simulink model "gm_hybrid_lht_vnl"  (R2019b)
settings: Solver=FixedStepDiscrete  StartTime=0.0  StopTime=inf  FixedStep=1/120e6  RelTol=1e-3
undefined symbols (not defined in the file or in its folder): bt, height, nTheta, width
libraries: hdlsllib x252, simulink x168, hdlmdlgenlib x11, dspsrcs4 x1
(part 8 of 12)

== system gm_hybrid_lht_vnl/Hybrid LHT/Hybrid LHT Kernel/Gradient Kernel System/Get Index and Fix Limits/GetShift1_instance25 ==
  Theta : Inport  OutDataTypeStr=uint8  PortDimensions=1  SampleTime=8.33333333333333e-09
  Add : Sum  Inputs=+  OutDataTypeStr=fixdt(0, ceil(log2(L+1)), 0)
  Constant : Constant  Value=U  VectorParams1D=off  OutDataTypeStr=fixdt(0,ceil(log2(max(U)+1)),0)  SampleTime=-1
  Relational Operator : RelationalOperator  OutDataTypeStr=boolean  RndMeth=Nearest
  Shift : Outport  VectorParamsAs1DForOutWhenUnconnected=off
  wires:
  Relational Operator/1 -> Add/1
  Constant/1 -> Relational Operator/2
  Add/1 -> Shift/1
  Theta/1 -> Relational Operator/1

== system gm_hybrid_lht_vnl/Hybrid LHT/Hybrid LHT Kernel/Gradient Kernel System/Get Index and Fix Limits/GetShift1_instance26 ==
  Theta : Inport  OutDataTypeStr=uint8  PortDimensions=1  SampleTime=8.33333333333333e-09
  Add : Sum  Inputs=+  OutDataTypeStr=fixdt(0, ceil(log2(L+1)), 0)
  Constant : Constant  Value=U  VectorParams1D=off  OutDataTypeStr=fixdt(0,ceil(log2(max(U)+1)),0)  SampleTime=-1
  Relational Operator : RelationalOperator  OutDataTypeStr=boolean  RndMeth=Nearest
  Shift : Outport  VectorParamsAs1DForOutWhenUnconnected=off
  wires:
  Relational Operator/1 -> Add/1
  Constant/1 -> Relational Operator/2
  Add/1 -> Shift/1
  Theta/1 -> Relational Operator/1

== system gm_hybrid_lht_vnl/Hybrid LHT/Hybrid LHT Kernel/Gradient Kernel System/Get Index and Fix Limits/GetShift1_instance27 ==
  Theta : Inport  OutDataTypeStr=uint8  PortDimensions=1  SampleTime=8.33333333333333e-09
  Add : Sum  Inputs=+  OutDataTypeStr=fixdt(0, ceil(log2(L+1)), 0)
  Constant : Constant  Value=U  VectorParams1D=off  OutDataTypeStr=fixdt(0,ceil(log2(max(U)+1)),0)  SampleTime=-1
  Relational Operator : RelationalOperator  OutDataTypeStr=boolean  RndMeth=Nearest
  Shift : Outport  VectorParamsAs1DForOutWhenUnconnected=off
  wires:
  Relational Operator/1 -> Add/1
  Constant/1 -> Relational Operator/2
  Add/1 -> Shift/1
  Theta/1 -> Relational Operator/1

== system gm_hybrid_lht_vnl/Hybrid LHT/Hybrid LHT Kernel/Gradient Kernel System/Get Index and Fix Limits/GetShift1_instance28 ==
  Theta : Inport  OutDataTypeStr=uint8  PortDimensions=1  SampleTime=8.33333333333333e-09
  Add : Sum  Inputs=+  OutDataTypeStr=fixdt(0, ceil(log2(L+1)), 0)
  Constant : Constant  Value=U  VectorParams1D=off  OutDataTypeStr=fixdt(0,ceil(log2(max(U)+1)),0)  SampleTime=-1
  Relational Operator : RelationalOperator  OutDataTypeStr=boolean  RndMeth=Nearest
  Shift : Outport  VectorParamsAs1DForOutWhenUnconnected=off
  wires:
  Relational Operator/1 -> Add/1
  Constant/1 -> Relational Operator/2
  Add/1 -> Shift/1
  Theta/1 -> Relational Operator/1

== system gm_hybrid_lht_vnl/Hybrid LHT/Hybrid LHT Kernel/Gradient Kernel System/Get Index and Fix Limits/GetShift1_instance29 ==
  Theta : Inport  OutDataTypeStr=uint8  PortDimensions=1  SampleTime=8.33333333333333e-09
  Add : Sum  Inputs=+  OutDataTypeStr=fixdt(0, ceil(log2(L+1)), 0)
  Constant : Constant  Value=U  VectorParams1D=off  OutDataTypeStr=fixdt(0,ceil(log2(max(U)+1)),0)  SampleTime=-1
  Relational Operator : RelationalOperator  OutDataTypeStr=boolean  RndMeth=Nearest
  Shift : Outport  VectorParamsAs1DForOutWhenUnconnected=off
  wires:
  Relational Operator/1 -> Add/1
  Constant/1 -> Relational Operator/2
  Add/1 -> Shift/1
  Theta/1 -> Relational Operator/1

== system gm_hybrid_lht_vnl/Hybrid LHT/Hybrid LHT Kernel/Gradient Kernel System/Get Index and Fix Limits/GetShift1_instance3 ==
  Theta : Inport  OutDataTypeStr=uint8  PortDimensions=1  SampleTime=8.33333333333333e-09
  Add : Sum  Inputs=+  OutDataTypeStr=fixdt(0, ceil(log2(L+1)), 0)
  Constant : Constant  Value=U  VectorParams1D=off  OutDataTypeStr=fixdt(0,ceil(log2(max(U)+1)),0)  SampleTime=-1
  Relational Operator : RelationalOperator  OutDataTypeStr=boolean  RndMeth=Nearest
  Shift : Outport  VectorParamsAs1DForOutWhenUnconnected=off
  wires:
  Relational Operator/1 -> Add/1
  Constant/1 -> Relational Operator/2
  Add/1 -> Shift/1
  Theta/1 -> Relational Operator/1

== system gm_hybrid_lht_vnl/Hybrid LHT/Hybrid LHT Kernel/Gradient Kernel System/Get Index and Fix Limits/GetShift1_instance30 ==
  Theta : Inport  OutDataTypeStr=uint8  PortDimensions=1  SampleTime=8.33333333333333e-09
  Add : Sum  Inputs=+  OutDataTypeStr=fixdt(0, ceil(log2(L+1)), 0)
  Constant : Constant  Value=U  VectorParams1D=off  OutDataTypeStr=fixdt(0,ceil(log2(max(U)+1)),0)  SampleTime=-1
  Relational Operator : RelationalOperator  OutDataTypeStr=boolean  RndMeth=Nearest
  Shift : Outport  VectorParamsAs1DForOutWhenUnconnected=off
  wires:
  Relational Operator/1 -> Add/1
  Constant/1 -> Relational Operator/2
  Add/1 -> Shift/1
  Theta/1 -> Relational Operator/1

== system gm_hybrid_lht_vnl/Hybrid LHT/Hybrid LHT Kernel/Gradient Kernel System/Get Index and Fix Limits/GetShift1_instance31 ==
  Theta : Inport  OutDataTypeStr=uint8  PortDimensions=1  SampleTime=8.33333333333333e-09
  Add : Sum  Inputs=+  OutDataTypeStr=fixdt(0, ceil(log2(L+1)), 0)
  Constant : Constant  Value=U  VectorParams1D=off  OutDataTypeStr=fixdt(0,ceil(log2(max(U)+1)),0)  SampleTime=-1
  Relational Operator : RelationalOperator  OutDataTypeStr=boolean  RndMeth=Nearest
  Shift : Outport  VectorParamsAs1DForOutWhenUnconnected=off
  wires:
  Relational Operator/1 -> Add/1
  Constant/1 -> Relational Operator/2
  Add/1 -> Shift/1
  Theta/1 -> Relational Operator/1

== system gm_hybrid_lht_vnl/Hybrid LHT/Hybrid LHT Kernel/Gradient Kernel System/Get Index and Fix Limits/GetShift1_instance32 ==
  Theta : Inport  OutDataTypeStr=uint8  PortDimensions=1  SampleTime=8.33333333333333e-09
  Add : Sum  Inputs=+  OutDataTypeStr=fixdt(0, ceil(log2(L+1)), 0)
  Constant : Constant  Value=U  VectorParams1D=off  OutDataTypeStr=fixdt(0,ceil(log2(max(U)+1)),0)  SampleTime=-1
  Relational Operator : RelationalOperator  OutDataTypeStr=boolean  RndMeth=Nearest
  Shift : Outport  VectorParamsAs1DForOutWhenUnconnected=off
  wires:
  Relational Operator/1 -> Add/1
  Constant/1 -> Relational Operator/2
  Add/1 -> Shift/1
  Theta/1 -> Relational Operator/1

== system gm_hybrid_lht_vnl/Hybrid LHT/Hybrid LHT Kernel/Gradient Kernel System/Get Index and Fix Limits/GetShift1_instance33 ==
  Theta : Inport  OutDataTypeStr=uint8  PortDimensions=1  SampleTime=8.33333333333333e-09
  Add : Sum  Inputs=+  OutDataTypeStr=fixdt(0, ceil(log2(L+1)), 0)
  Constant : Constant  Value=U  VectorParams1D=off  OutDataTypeStr=fixdt(0,ceil(log2(max(U)+1)),0)  SampleTime=-1
  Relational Operator : RelationalOperator  OutDataTypeStr=boolean  RndMeth=Nearest
  Shift : Outport  VectorParamsAs1DForOutWhenUnconnected=off
  wires:
  Relational Operator/1 -> Add/1
  Constant/1 -> Relational Operator/2
  Add/1 -> Shift/1
  Theta/1 -> Relational Operator/1

== system gm_hybrid_lht_vnl/Hybrid LHT/Hybrid LHT Kernel/Gradient Kernel System/Get Index and Fix Limits/GetShift1_instance34 ==
  Theta : Inport  OutDataTypeStr=uint8  PortDimensions=1  SampleTime=8.33333333333333e-09
  Add : Sum  Inputs=+  OutDataTypeStr=fixdt(0, ceil(log2(L+1)), 0)
  Constant : Constant  Value=U  VectorParams1D=off  OutDataTypeStr=fixdt(0,ceil(log2(max(U)+1)),0)  SampleTime=-1
  Relational Operator : RelationalOperator  OutDataTypeStr=boolean  RndMeth=Nearest
  Shift : Outport  VectorParamsAs1DForOutWhenUnconnected=off
  wires:
  Relational Operator/1 -> Add/1
  Constant/1 -> Relational Operator/2
  Add/1 -> Shift/1
  Theta/1 -> Relational Operator/1

== system gm_hybrid_lht_vnl/Hybrid LHT/Hybrid LHT Kernel/Gradient Kernel System/Get Index and Fix Limits/GetShift1_instance35 ==
  Theta : Inport  OutDataTypeStr=uint8  PortDimensions=1  SampleTime=8.33333333333333e-09
  Add : Sum  Inputs=+  OutDataTypeStr=fixdt(0, ceil(log2(L+1)), 0)
  Constant : Constant  Value=U  VectorParams1D=off  OutDataTypeStr=fixdt(0,ceil(log2(max(U)+1)),0)  SampleTime=-1
  Relational Operator : RelationalOperator  OutDataTypeStr=boolean  RndMeth=Nearest
  Shift : Outport  VectorParamsAs1DForOutWhenUnconnected=off
  wires:
  Relational Operator/1 -> Add/1
  Constant/1 -> Relational Operator/2
  Add/1 -> Shift/1
  Theta/1 -> Relational Operator/1

== system gm_hybrid_lht_vnl/Hybrid LHT/Hybrid LHT Kernel/Gradient Kernel System/Get Index and Fix Limits/GetShift1_instance36 ==
  Theta : Inport  OutDataTypeStr=uint8  PortDimensions=1  SampleTime=8.33333333333333e-09
  Add : Sum  Inputs=+  OutDataTypeStr=fixdt(0, ceil(log2(L+1)), 0)
  Constant : Constant  Value=U  VectorParams1D=off  OutDataTypeStr=fixdt(0,ceil(log2(max(U)+1)),0)  SampleTime=-1
  Relational Operator : RelationalOperator  OutDataTypeStr=boolean  RndMeth=Nearest
  Shift : Outport  VectorParamsAs1DForOutWhenUnconnected=off
  wires:
  Relational Operator/1 -> Add/1
  Constant/1 -> Relational Operator/2
  Add/1 -> Shift/1
  Theta/1 -> Relational Operator/1

== system gm_hybrid_lht_vnl/Hybrid LHT/Hybrid LHT Kernel/Gradient Kernel System/Get Index and Fix Limits/GetShift1_instance37 ==
  Theta : Inport  OutDataTypeStr=uint8  PortDimensions=1  SampleTime=8.33333333333333e-09
  Add : Sum  Inputs=+  OutDataTypeStr=fixdt(0, ceil(log2(L+1)), 0)
  Constant : Constant  Value=U  VectorParams1D=off  OutDataTypeStr=fixdt(0,ceil(log2(max(U)+1)),0)  SampleTime=-1
  Relational Operator : RelationalOperator  OutDataTypeStr=boolean  RndMeth=Nearest
  Shift : Outport  VectorParamsAs1DForOutWhenUnconnected=off
  wires:
  Relational Operator/1 -> Add/1
  Constant/1 -> Relational Operator/2
  Add/1 -> Shift/1
  Theta/1 -> Relational Operator/1

== system gm_hybrid_lht_vnl/Hybrid LHT/Hybrid LHT Kernel/Gradient Kernel System/Get Index and Fix Limits/GetShift1_instance38 ==
  Theta : Inport  OutDataTypeStr=uint8  PortDimensions=1  SampleTime=8.33333333333333e-09
  Add : Sum  Inputs=+  OutDataTypeStr=fixdt(0, ceil(log2(L+1)), 0)
  Constant : Constant  Value=U  VectorParams1D=off  OutDataTypeStr=fixdt(0,ceil(log2(max(U)+1)),0)  SampleTime=-1
  Relational Operator : RelationalOperator  OutDataTypeStr=boolean  RndMeth=Nearest
  Shift : Outport  VectorParamsAs1DForOutWhenUnconnected=off
  wires:
  Relational Operator/1 -> Add/1
  Constant/1 -> Relational Operator/2
  Add/1 -> Shift/1
  Theta/1 -> Relational Operator/1

== system gm_hybrid_lht_vnl/Hybrid LHT/Hybrid LHT Kernel/Gradient Kernel System/Get Index and Fix Limits/GetShift1_instance39 ==
  Theta : Inport  OutDataTypeStr=uint8  PortDimensions=1  SampleTime=8.33333333333333e-09
  Add : Sum  Inputs=+  OutDataTypeStr=fixdt(0, ceil(log2(L+1)), 0)
  Constant : Constant  Value=U  VectorParams1D=off  OutDataTypeStr=fixdt(0,ceil(log2(max(U)+1)),0)  SampleTime=-1
  Relational Operator : RelationalOperator  OutDataTypeStr=boolean  RndMeth=Nearest
  Shift : Outport  VectorParamsAs1DForOutWhenUnconnected=off
  wires:
  Relational Operator/1 -> Add/1
  Constant/1 -> Relational Operator/2
  Add/1 -> Shift/1
  Theta/1 -> Relational Operator/1

== system gm_hybrid_lht_vnl/Hybrid LHT/Hybrid LHT Kernel/Gradient Kernel System/Get Index and Fix Limits/GetShift1_instance4 ==
  Theta : Inport  OutDataTypeStr=uint8  PortDimensions=1  SampleTime=8.33333333333333e-09
  Add : Sum  Inputs=+  OutDataTypeStr=fixdt(0, ceil(log2(L+1)), 0)
  Constant : Constant  Value=U  VectorParams1D=off  OutDataTypeStr=fixdt(0,ceil(log2(max(U)+1)),0)  SampleTime=-1
  Relational Operator : RelationalOperator  OutDataTypeStr=boolean  RndMeth=Nearest
  Shift : Outport  VectorParamsAs1DForOutWhenUnconnected=off
  wires:
  Relational Operator/1 -> Add/1
  Constant/1 -> Relational Operator/2
  Add/1 -> Shift/1
  Theta/1 -> Relational Operator/1

== system gm_hybrid_lht_vnl/Hybrid LHT/Hybrid LHT Kernel/Gradient Kernel System/Get Index and Fix Limits/GetShift1_instance40 ==
  Theta : Inport  OutDataTypeStr=uint8  PortDimensions=1  SampleTime=8.33333333333333e-09
  Add : Sum  Inputs=+  OutDataTypeStr=fixdt(0, ceil(log2(L+1)), 0)
  Constant : Constant  Value=U  VectorParams1D=off  OutDataTypeStr=fixdt(0,ceil(log2(max(U)+1)),0)  SampleTime=-1
  Relational Operator : RelationalOperator  OutDataTypeStr=boolean  RndMeth=Nearest
  Shift : Outport  VectorParamsAs1DForOutWhenUnconnected=off
  wires:
  Relational Operator/1 -> Add/1
  Constant/1 -> Relational Operator/2
  Add/1 -> Shift/1
  Theta/1 -> Relational Operator/1

== system gm_hybrid_lht_vnl/Hybrid LHT/Hybrid LHT Kernel/Gradient Kernel System/Get Index and Fix Limits/GetShift1_instance41 ==
  Theta : Inport  OutDataTypeStr=uint8  PortDimensions=1  SampleTime=8.33333333333333e-09
  Add : Sum  Inputs=+  OutDataTypeStr=fixdt(0, ceil(log2(L+1)), 0)
  Constant : Constant  Value=U  VectorParams1D=off  OutDataTypeStr=fixdt(0,ceil(log2(max(U)+1)),0)  SampleTime=-1
  Relational Operator : RelationalOperator  OutDataTypeStr=boolean  RndMeth=Nearest
  Shift : Outport  VectorParamsAs1DForOutWhenUnconnected=off
  wires:
  Relational Operator/1 -> Add/1
  Constant/1 -> Relational Operator/2
  Add/1 -> Shift/1
  Theta/1 -> Relational Operator/1

== system gm_hybrid_lht_vnl/Hybrid LHT/Hybrid LHT Kernel/Gradient Kernel System/Get Index and Fix Limits/GetShift1_instance42 ==
  Theta : Inport  OutDataTypeStr=uint8  PortDimensions=1  SampleTime=8.33333333333333e-09
  Add : Sum  Inputs=+  OutDataTypeStr=fixdt(0, ceil(log2(L+1)), 0)
  Constant : Constant  Value=U  VectorParams1D=off  OutDataTypeStr=fixdt(0,ceil(log2(max(U)+1)),0)  SampleTime=-1
  Relational Operator : RelationalOperator  OutDataTypeStr=boolean  RndMeth=Nearest
  Shift : Outport  VectorParamsAs1DForOutWhenUnconnected=off
  wires:
  Relational Operator/1 -> Add/1
  Constant/1 -> Relational Operator/2
  Add/1 -> Shift/1
  Theta/1 -> Relational Operator/1

== system gm_hybrid_lht_vnl/Hybrid LHT/Hybrid LHT Kernel/Gradient Kernel System/Get Index and Fix Limits/GetShift1_instance43 ==
  Theta : Inport  OutDataTypeStr=uint8  PortDimensions=1  SampleTime=8.33333333333333e-09
  Add : Sum  Inputs=+  OutDataTypeStr=fixdt(0, ceil(log2(L+1)), 0)
  Constant : Constant  Value=U  VectorParams1D=off  OutDataTypeStr=fixdt(0,ceil(log2(max(U)+1)),0)  SampleTime=-1
  Relational Operator : RelationalOperator  OutDataTypeStr=boolean  RndMeth=Nearest
  Shift : Outport  VectorParamsAs1DForOutWhenUnconnected=off
  wires:
  Relational Operator/1 -> Add/1
  Constant/1 -> Relational Operator/2
  Add/1 -> Shift/1
  Theta/1 -> Relational Operator/1

== system gm_hybrid_lht_vnl/Hybrid LHT/Hybrid LHT Kernel/Gradient Kernel System/Get Index and Fix Limits/GetShift1_instance44 ==
  Theta : Inport  OutDataTypeStr=uint8  PortDimensions=1  SampleTime=8.33333333333333e-09
  Add : Sum  Inputs=+  OutDataTypeStr=fixdt(0, ceil(log2(L+1)), 0)
  Constant : Constant  Value=U  VectorParams1D=off  OutDataTypeStr=fixdt(0,ceil(log2(max(U)+1)),0)  SampleTime=-1
  Relational Operator : RelationalOperator  OutDataTypeStr=boolean  RndMeth=Nearest
  Shift : Outport  VectorParamsAs1DForOutWhenUnconnected=off
  wires:
  Relational Operator/1 -> Add/1
  Constant/1 -> Relational Operator/2
  Add/1 -> Shift/1
  Theta/1 -> Relational Operator/1

== system gm_hybrid_lht_vnl/Hybrid LHT/Hybrid LHT Kernel/Gradient Kernel System/Get Index and Fix Limits/GetShift1_instance45 ==
  Theta : Inport  OutDataTypeStr=uint8  PortDimensions=1  SampleTime=8.33333333333333e-09
  Add : Sum  Inputs=+  OutDataTypeStr=fixdt(0, ceil(log2(L+1)), 0)
  Constant : Constant  Value=U  VectorParams1D=off  OutDataTypeStr=fixdt(0,ceil(log2(max(U)+1)),0)  SampleTime=-1
  Relational Operator : RelationalOperator  OutDataTypeStr=boolean  RndMeth=Nearest
  Shift : Outport  VectorParamsAs1DForOutWhenUnconnected=off
  wires:
  Relational Operator/1 -> Add/1
  Constant/1 -> Relational Operator/2
  Add/1 -> Shift/1
  Theta/1 -> Relational Operator/1

== system gm_hybrid_lht_vnl/Hybrid LHT/Hybrid LHT Kernel/Gradient Kernel System/Get Index and Fix Limits/GetShift1_instance5 ==
  Theta : Inport  OutDataTypeStr=uint8  PortDimensions=1  SampleTime=8.33333333333333e-09
  Add : Sum  Inputs=+  OutDataTypeStr=fixdt(0, ceil(log2(L+1)), 0)
  Constant : Constant  Value=U  VectorParams1D=off  OutDataTypeStr=fixdt(0,ceil(log2(max(U)+1)),0)  SampleTime=-1
  Relational Operator : RelationalOperator  OutDataTypeStr=boolean  RndMeth=Nearest
  Shift : Outport  VectorParamsAs1DForOutWhenUnconnected=off
  wires:
  Relational Operator/1 -> Add/1
  Constant/1 -> Relational Operator/2
  Add/1 -> Shift/1
  Theta/1 -> Relational Operator/1

== system gm_hybrid_lht_vnl/Hybrid LHT/Hybrid LHT Kernel/Gradient Kernel System/Get Index and Fix Limits/GetShift1_instance6 ==
  Theta : Inport  OutDataTypeStr=uint8  PortDimensions=1  SampleTime=8.33333333333333e-09
  Add : Sum  Inputs=+  OutDataTypeStr=fixdt(0, ceil(log2(L+1)), 0)
  Constant : Constant  Value=U  VectorParams1D=off  OutDataTypeStr=fixdt(0,ceil(log2(max(U)+1)),0)  SampleTime=-1
  Relational Operator : RelationalOperator  OutDataTypeStr=boolean  RndMeth=Nearest
  Shift : Outport  VectorParamsAs1DForOutWhenUnconnected=off
  wires:
  Relational Operator/1 -> Add/1
  Constant/1 -> Relational Operator/2
  Add/1 -> Shift/1
  Theta/1 -> Relational Operator/1

== system gm_hybrid_lht_vnl/Hybrid LHT/Hybrid LHT Kernel/Gradient Kernel System/Get Index and Fix Limits/GetShift1_instance7 ==
  Theta : Inport  OutDataTypeStr=uint8  PortDimensions=1  SampleTime=8.33333333333333e-09
  Add : Sum  Inputs=+  OutDataTypeStr=fixdt(0, ceil(log2(L+1)), 0)
  Constant : Constant  Value=U  VectorParams1D=off  OutDataTypeStr=fixdt(0,ceil(log2(max(U)+1)),0)  SampleTime=-1
  Relational Operator : RelationalOperator  OutDataTypeStr=boolean  RndMeth=Nearest
  Shift : Outport  VectorParamsAs1DForOutWhenUnconnected=off
  wires:
  Relational Operator/1 -> Add/1
  Constant/1 -> Relational Operator/2
  Add/1 -> Shift/1
  Theta/1 -> Relational Operator/1

== system gm_hybrid_lht_vnl/Hybrid LHT/Hybrid LHT Kernel/Gradient Kernel System/Get Index and Fix Limits/GetShift1_instance8 ==
  Theta : Inport  OutDataTypeStr=uint8  PortDimensions=1  SampleTime=8.33333333333333e-09
  Add : Sum  Inputs=+  OutDataTypeStr=fixdt(0, ceil(log2(L+1)), 0)
  Constant : Constant  Value=U  VectorParams1D=off  OutDataTypeStr=fixdt(0,ceil(log2(max(U)+1)),0)  SampleTime=-1
  Relational Operator : RelationalOperator  OutDataTypeStr=boolean  RndMeth=Nearest
  Shift : Outport  VectorParamsAs1DForOutWhenUnconnected=off
  wires:
  Relational Operator/1 -> Add/1
  Constant/1 -> Relational Operator/2
  Add/1 -> Shift/1
  Theta/1 -> Relational Operator/1

== system gm_hybrid_lht_vnl/Hybrid LHT/Hybrid LHT Kernel/Gradient Kernel System/Get Index and Fix Limits/GetShift1_instance9 ==
  Theta : Inport  OutDataTypeStr=uint8  PortDimensions=1  SampleTime=8.33333333333333e-09
  Add : Sum  Inputs=+  OutDataTypeStr=fixdt(0, ceil(log2(L+1)), 0)
  Constant : Constant  Value=U  VectorParams1D=off  OutDataTypeStr=fixdt(0,ceil(log2(max(U)+1)),0)  SampleTime=-1
  Relational Operator : RelationalOperator  OutDataTypeStr=boolean  RndMeth=Nearest
  Shift : Outport  VectorParamsAs1DForOutWhenUnconnected=off
  wires:
  Relational Operator/1 -> Add/1
  Constant/1 -> Relational Operator/2
  Add/1 -> Shift/1
  Theta/1 -> Relational Operator/1

== system gm_hybrid_lht_vnl/Hybrid LHT/Hybrid LHT Kernel/Gradient Kernel System/Hough Kernel/Hough Kernel ==
  X : Inport  OutDataTypeStr=fixdt(1, 9, 0)  PortDimensions=1  SampleTime=8.33333333333333e-09
  Y : Inport  Port=2  OutDataTypeStr=int8  PortDimensions=[1 180]  SampleTime=8.33333333333333e-09
  Index : Inport  Port=3  OutDataTypeStr=uint8  PortDimensions=[1 45]  SampleTime=8.33333333333333e-09
  Add : Sum  AccumDataTypeStr=fixdt(1, 10, 0)  OutDataTypeStr=fixdt(1, 9, 0)  RndMeth=Round  SampleTime=8.33333333333333e-09
  CosineROM : Constant  Value=[1 0.9998779296875 0.9993896484375 0.9986572265625 0.99755859375 0.9962158203125 0.9945068359375 0.9925537109375 0.99029541015625 0.9876708984375 0.98480224609375 0.98162841796875 0.9781494140625 0.974365234375 0.97027587890625 0.9659423828125 0.96124267578125 0.956298828125 0.9510498046875 0.94549560546875 0.939697265625 0.93359375 0.92718505859375 0.9205322265625 0.91357421875 0.90631103515625 0.8988037109375 0.8909912109375 0.8829345703125 0.8746337890625 0.86602783203125 0.857177734375 0.8480224609375 0.83868408203125 0.82904052734375 0.81915283203125 0.80902099609375 0.79864501953125 0.78802490234375 0.77716064453125 0.76605224609375 0.75469970703125 0.7431640625 0.7313232421875 0.7193603515625 0.70709228515625 0.69464111328125 0.6820068359375 0.66912841796875 0.65606689453125 0.64276123046875 0.62933349609375 0.61566162109375 0.601806640625 0.5877685546875 0.57354736328125 0.5592041015625 0.54461669921875 0.5299072265625 0.5150146484375 0.5 0.48480224609375 0.469482421875 0.4539794921875 0.4383544921875 0.422607421875 0.40673828125 0.3907470703125 0.3746337890625 0.3583984375 0.342041015625 0.3255615234375 0.30902099609375 0.2923583984375 0.275634765625 0.2587890625 0.241943359375 0.2249755859375 0.2078857421875 0.1907958984375 0.17364501953125 0.15643310546875 0.13916015625 0.12188720703125 0.10455322265625 0.087158203125 0.06976318359375 0.05230712890625 0.034912109375 0.0174560546875 0 -0.0174560546875 -0.034912109375 -0.05230712890625 -0.06976318359375 -0.087158203125 -0.10455322265625 -0.12188720703125 -0.13916015625 -0.15643310546875 -0.17364501953125 -0.1907958984375 -0.2078857421875 -0.2249755859375 -0.241943359375 -0.2587890625 -0.275634765625 -0.2923583984375 -0.30902099609375 -0.3255615234375 -0.342041015625 -0.3583984375 -0.3746337890625 -0.3907470703125 -0.40673828125 -0.422607421875 -0.4383544921875 -0.4539794921875 -0.469482421875 -0.48480224609375 -0.5 -0.5150146484375 -0.5299072265625 -0.54461669921875 -0.5592041015625 -0.57354736328125 -0.5877685546875 -0.601806640625 -0.61566162109375 -0.62933349609375 -0.64276123046875 -0.65606689453125 -0.66912841796875 -0.6820068359375 -0.69464111328125 -0.70709228515625 -0.7193603515625 -0.7313232421875 -0.7431640625 -0.75469970703125 -0.76605224609375 -0.77716064453125 -0.78802490234375 -0.79864501953125 -0.80902099609375 -0.81915283203125 -0.82904052734375 -0.83868408203125 -0.8480224609375 -0.857177734375 -0.86602783203125 -0.8746337890625 -0.8829345703125 -0.8909912109375 -0.8988037109375 -0.90631103515625 -0.91357421875 -0.9205322265625 -0.92718505859375 -0.93359375 -0.939697265625 -0.94549560546875 -0.9510498046875 -0.956298828125 -0.96124267578125 -0.9659423828125 -0.97027587890625 -0.974365234375 -0.9781494140625 -0.98162841796875 -0.98480224609375 -0.9876708984375 -0.99029541015625 -0.9925537109375 -0.9945068359375 -0.9962158203125 -0.99755859375 -0.9986572265625 -0.9993896484375 -0.9998779296875]  VectorParams1D=off  OutDataTypeStr=fixdt(1, 16, 14)  SampleTime=-1
  HwModeRegister : Delay  DelayLength=double(1)  InitialCondition=0  SampleTime=8.33333333333333e-09
  HwModeRegister1 : Delay  DelayLength=double(1)  InitialCondition=0  SampleTime=8.33333333333333e-09
  PipelineRegister : Delay  DelayLength=double(1)  InitialCondition=0  SampleTime=8.33333333333333e-09
  Selector : Selector  NumberOfDimensions=2  IndexMode=Zero-based  SampleTime=8.33333333333333e-09  IndexOptions=Index vector (dialog),Index vector (port)  Indices=double(0),double(1)  OutputSizes=double(1),double(1)
  Selector1 : Selector  NumberOfDimensions=2  IndexMode=Zero-based  SampleTime=8.33333333333333e-09  IndexOptions=Index vector (dialog),Index vector (port)  Indices=double(0),double(1)  OutputSizes=double(1),double(1)
  delayMatch : Delay  DelayLength=double(2)  InitialCondition=0  SampleTime=8.33333333333333e-09
  xcos : Product  Inputs=**  OutDataTypeStr=fixdt(1, 25, 14)  SampleTime=8.33333333333333e-09
  xcos_in0_buff : hdlmdlgenlib/Buffer
      settings: SourceProductName=Simulink  SourceProductBaseCode=SL
  xcos_in1_buff : hdlmdlgenlib/Buffer
      settings: SourceProductName=Simulink  SourceProductBaseCode=SL
  xcos_out_dtc : DataTypeConversion  OutDataTypeStr=fixdt(1, 9, 0)  RndMeth=Round  SampleTime=8.33333333333333e-09
  Rho : Outport  VectorParamsAs1DForOutWhenUnconnected=off
  wires:
  xcos_in1_buff/1 -> HwModeRegister1/1
  xcos_in0_buff/1 -> HwModeRegister/1
  HwModeRegister1/1 -> xcos/2
  HwModeRegister/1 -> xcos/1
  xcos/1 -> PipelineRegister/1
  Index/1 -> Selector/2, delayMatch/1
  Y/1 -> Selector1/1
  X/1 -> xcos_in0_buff/1
  PipelineRegister/1 -> xcos_out_dtc/1
  xcos_out_dtc/1 -> Add/1
  Selector1/1 -> Add/2
  Selector/1 -> xcos_in1_buff/1
  CosineROM/1 -> Selector/1
  Add/1 -> Rho/1
  delayMatch/1 -> Selector1/2

== system gm_hybrid_lht_vnl/Hybrid LHT/Hybrid LHT Kernel/Gradient Kernel System/Hough Kernel/Look Ahead Hough ==
  Y : Inport  OutDataTypeStr=int8  PortDimensions=1  SampleTime=8.33333333333333e-09
  eol : Inport  Port=2  OutDataTypeStr=boolean  PortDimensions=1  SampleTime=8.33333333333333e-09
  Look Ahead Hough Symmetric : Subsystem
  ysin : Outport
  wires:
  eol/1 -> Look Ahead Hough Symmetric/2(eol)
  Y/1 -> Look Ahead Hough Symmetric/1(Y)
  Look Ahead Hough Symmetric/1(ysin) -> ysin/1

== system gm_hybrid_lht_vnl/Hybrid LHT_vnl/Hybrid LHT Accumulator/Accumulator with Switches/Accumulator/Block RAM ==
  wr_data : Inport
  wr_addr : Inport  Port=2
  wr_en : Inport  Port=3
  rd_addr : Inport  Port=4
  Simple Dual Port RAM : Subsystem  VariantControl=9_bits
  Simple Dual Port RAM Generator : Subsystem  VariantControl=other_bits  mask{b=36, d=400, b_hidden=36, d_hidden=400}
      mask prompts: b "Data width:"; d "Depth:"
      mask init: same as gm_hybrid_lht_vnl/Hybrid LHT/Hybrid LHT Accumulator/Accumulator with Switches/Accumulator_instance1/Block RAM/Simple Dual Port RAM Generator
  rd_data : Outport

== system gm_hybrid_lht_vnl/Hybrid LHT_vnl/Hybrid LHT Kernel/Gradient Kernel System/Get Index and Fix Limits/Extract Active Votes ==
  note: Check the indices to ensure they are in the correct limits
  Theta : Inport
  Add : Sum
  Add1 : Sum  Inputs=+-
  Add3 : Sum
  Constant : Constant  Value=[-lambda:1:lambda-subflag]  VectorParams1D=off  OutDataTypeStr=fixdt(1,ceil(log2(lambda+1))+1, 0)  SampleTime=-1
  Data Type Conversion : DataTypeConversion  OutDataTypeStr=fixdt(0, ceil(log2(nTheta+1)), 0)
  High : Constant  Value=nTheta-1  OutDataTypeStr=fixdt(0,ceil(log2(nTheta)),0)  SampleTime=-1
  Low : Constant  Value=0  OutDataTypeStr=fixdt(0,1,0)  SampleTime=-1
  Multiport Switch2 : MultiPortSwitch  DataPortOrder=Zero-based contiguous  Inputs=2  zeroidx=on
  Multiport Switch3 : MultiPortSwitch  DataPortOrder=Zero-based contiguous  Inputs=2  zeroidx=on
  Relational : RelationalOperator  Operator=<  OutDataTypeStr=boolean  RndMeth=Nearest
  Relational1 : RelationalOperator  Operator=>  OutDataTypeStr=boolean  RndMeth=Nearest
  nTheta : Constant  Value=nTheta  OutDataTypeStr=fixdt(0,ceil(log2(nTheta+1)),0)  SampleTime=-1
  Index : Outport  VectorParamsAs1DForOutWhenUnconnected=off
  wires:
  Data Type Conversion/1 -> Index/1
  Theta/1 -> Add/1
  Add/1 -> Multiport Switch2/2, Relational/1, Add3/1
  nTheta/1 -> Add1/2, Add3/2
  Multiport Switch2/1 -> Multiport Switch3/2, Relational1/1, Add1/1
  Low/1 -> Relational/2
  Add3/1 -> Multiport Switch2/3
  Relational1/1 -> Multiport Switch3/1
  High/1 -> Relational1/2
  Multiport Switch3/1 -> Data Type Conversion/1
  Relational/1 -> Multiport Switch2/1
  Add1/1 -> Multiport Switch3/3
  Constant/1 -> Add/2

== system gm_hybrid_lht_vnl/Hybrid LHT_vnl/Hybrid LHT Kernel/Gradient Kernel System/Get Index and Fix Limits/GetShift1 ==
  Theta : Inport  Partition=on  PartitionDimension=2  PartitionWidth=1  PartitionOffset=0
  Add : Sum  Inputs=+  OutDataTypeStr=fixdt(0, ceil(log2(L+1)), 0)
  Constant : Constant  Value=U  VectorParams1D=off  OutDataTypeStr=fixdt(0,ceil(log2(max(U)+1)),0)  SampleTime=-1
  For Each : ForEach  DisableCoverage=on
  Relational Operator : RelationalOperator  OutDataTypeStr=boolean  RndMeth=Nearest
  Shift : Outport  ConcatenationDimension=2  VectorParamsAs1DForOutWhenUnconnected=off
  wires:
  Relational Operator/1 -> Add/1
  Add/1 -> Shift/1
  Theta/1 -> Relational Operator/1
  Constant/1 -> Relational Operator/2

== system gm_hybrid_lht_vnl/Hybrid LHT_vnl/Hybrid LHT Kernel/Gradient Kernel System/Hough Kernel/Hough Kernel ==
  X : Inport
  Y : Inport  Port=2
  Index : Inport  Port=3
  Add : Sum  OutDataTypeStr=fixdt(1, ceil(log2(2*maxRho)), 0)  RndMeth=Round
  CosineROM : Constant  Value=fi(cos(deg2rad(theta)), 1, 16, 14)  VectorParams1D=off  OutDataTypeStr=fixdt(1,16,14)  SampleTime=-1
  Selector : Selector  NumberOfDimensions=2  IndexMode=Zero-based  InputPortWidth=3  IndexOptions=Index vector (dialog),Index vector (port)  Indices=0,1  OutputSizes=1,1
  Selector1 : Selector  NumberOfDimensions=2  IndexMode=Zero-based  InputPortWidth=3  IndexOptions=Index vector (dialog),Index vector (port)  Indices=0,1  OutputSizes=1,1
  xcos : Product  OutDataTypeStr=fixdt(1, ceil(log2(width+1)), 0);  RndMeth=Round
  Rho : Outport  VectorParamsAs1DForOutWhenUnconnected=off
  wires:
  Selector1/1 -> Add/2
  Y/1 -> Selector1/1
  CosineROM/1 -> Selector/1
  Selector/1 -> xcos/2
  xcos/1 -> Add/1
  Add/1 -> Rho/1
  X/1 -> xcos/1
  Index/1 -> Selector/2, Selector1/2

== system gm_hybrid_lht_vnl/Hybrid LHT_vnl/Hybrid LHT Kernel/Gradient Kernel System/Hough Kernel/Look Ahead Hough ==
  Y : Inport
  eol : Inport  Port=2
  Look Ahead Hough : Subsystem  VariantControl=Normal
  Look Ahead Hough Symmetric : Subsystem  VariantControl=Symmetric
  ysin : Outport

== system gm_hybrid_lht_vnl/Hybrid LHT/Hybrid LHT Accumulator/Accumulator with Switches/Accumulator_instance1/Block RAM/Simple Dual Port RAM Generator ==
  wr_data : Inport  OutDataTypeStr=fixdt(0, 36, 0)  PortDimensions=1  SampleTime=8.33333333333333e-09
  wr_addr : Inport  Port=2  OutDataTypeStr=fixdt(0, 9, 0)  PortDimensions=1  SampleTime=8.33333333333333e-09
  wr_en : Inport  Port=3  OutDataTypeStr=boolean  PortDimensions=1  SampleTime=8.33333333333333e-09
  rd_addr : Inport  Port=4  OutDataTypeStr=fixdt(0, 9, 0)  PortDimensions=1  SampleTime=8.33333333333333e-09
  rd_address : hdlsllib/Logic and Bit Operations/Bit Slice  lidx=8  ridx=0
      settings: SourceProductName=Simulink  SourceProductBaseCode=SL
  simple_ram_0 : hdlsllib/HDL RAMs/Simple Dual Port RAM  ram_size=9
      settings: SourceProductName=Simulink  SourceProductBaseCode=SL
  wr_address : hdlsllib/Logic and Bit Operations/Bit Slice  lidx=8  ridx=0
      settings: SourceProductName=Simulink  SourceProductBaseCode=SL
  rd_data : Outport
  wires:
  rd_addr/1 -> rd_address/1
  wr_en/1 -> simple_ram_0/3
  wr_addr/1 -> wr_address/1
  wr_data/1 -> simple_ram_0/1
  rd_address/1 -> simple_ram_0/4
  simple_ram_0/1 -> rd_data/1
  wr_address/1 -> simple_ram_0/2

== system gm_hybrid_lht_vnl/Hybrid LHT/Hybrid LHT Accumulator/Accumulator with Switches/Accumulator_instance10/Block RAM/Simple Dual Port RAM Generator ==
  wr_data : Inport  OutDataTypeStr=fixdt(0, 36, 0)  PortDimensions=1  SampleTime=8.33333333333333e-09
  wr_addr : Inport  Port=2  OutDataTypeStr=fixdt(0, 9, 0)  PortDimensions=1  SampleTime=8.33333333333333e-09
  wr_en : Inport  Port=3  OutDataTypeStr=boolean  PortDimensions=1  SampleTime=8.33333333333333e-09
  rd_addr : Inport  Port=4  OutDataTypeStr=fixdt(0, 9, 0)  PortDimensions=1  SampleTime=8.33333333333333e-09
  rd_address : hdlsllib/Logic and Bit Operations/Bit Slice  lidx=8  ridx=0
      settings: SourceProductName=Simulink  SourceProductBaseCode=SL
  simple_ram_0 : hdlsllib/HDL RAMs/Simple Dual Port RAM  ram_size=9
      settings: SourceProductName=Simulink  SourceProductBaseCode=SL
  wr_address : hdlsllib/Logic and Bit Operations/Bit Slice  lidx=8  ridx=0
      settings: SourceProductName=Simulink  SourceProductBaseCode=SL
  rd_data : Outport
  wires:
  wr_address/1 -> simple_ram_0/2
  simple_ram_0/1 -> rd_data/1
  rd_address/1 -> simple_ram_0/4
  wr_data/1 -> simple_ram_0/1
  wr_addr/1 -> wr_address/1
  wr_en/1 -> simple_ram_0/3
  rd_addr/1 -> rd_address/1

== system gm_hybrid_lht_vnl/Hybrid LHT/Hybrid LHT Accumulator/Accumulator with Switches/Accumulator_instance11/Block RAM/Simple Dual Port RAM Generator ==
  wr_data : Inport  OutDataTypeStr=fixdt(0, 36, 0)  PortDimensions=1  SampleTime=8.33333333333333e-09
  wr_addr : Inport  Port=2  OutDataTypeStr=fixdt(0, 9, 0)  PortDimensions=1  SampleTime=8.33333333333333e-09
  wr_en : Inport  Port=3  OutDataTypeStr=boolean  PortDimensions=1  SampleTime=8.33333333333333e-09
  rd_addr : Inport  Port=4  OutDataTypeStr=fixdt(0, 9, 0)  PortDimensions=1  SampleTime=8.33333333333333e-09
  rd_address : hdlsllib/Logic and Bit Operations/Bit Slice  lidx=8  ridx=0
      settings: SourceProductName=Simulink  SourceProductBaseCode=SL
  simple_ram_0 : hdlsllib/HDL RAMs/Simple Dual Port RAM  ram_size=9
      settings: SourceProductName=Simulink  SourceProductBaseCode=SL
  wr_address : hdlsllib/Logic and Bit Operations/Bit Slice  lidx=8  ridx=0
      settings: SourceProductName=Simulink  SourceProductBaseCode=SL
  rd_data : Outport
  wires:
  wr_address/1 -> simple_ram_0/2
  simple_ram_0/1 -> rd_data/1
  rd_address/1 -> simple_ram_0/4
  wr_data/1 -> simple_ram_0/1
  wr_addr/1 -> wr_address/1
  wr_en/1 -> simple_ram_0/3
  rd_addr/1 -> rd_address/1

== system gm_hybrid_lht_vnl/Hybrid LHT/Hybrid LHT Accumulator/Accumulator with Switches/Accumulator_instance12/Block RAM/Simple Dual Port RAM Generator ==
  wr_data : Inport  OutDataTypeStr=fixdt(0, 36, 0)  PortDimensions=1  SampleTime=8.33333333333333e-09
  wr_addr : Inport  Port=2  OutDataTypeStr=fixdt(0, 9, 0)  PortDimensions=1  SampleTime=8.33333333333333e-09
  wr_en : Inport  Port=3  OutDataTypeStr=boolean  PortDimensions=1  SampleTime=8.33333333333333e-09
  rd_addr : Inport  Port=4  OutDataTypeStr=fixdt(0, 9, 0)  PortDimensions=1  SampleTime=8.33333333333333e-09
  rd_address : hdlsllib/Logic and Bit Operations/Bit Slice  lidx=8  ridx=0
      settings: SourceProductName=Simulink  SourceProductBaseCode=SL
  simple_ram_0 : hdlsllib/HDL RAMs/Simple Dual Port RAM  ram_size=9
      settings: SourceProductName=Simulink  SourceProductBaseCode=SL
  wr_address : hdlsllib/Logic and Bit Operations/Bit Slice  lidx=8  ridx=0
      settings: SourceProductName=Simulink  SourceProductBaseCode=SL
  rd_data : Outport
  wires:
  wr_address/1 -> simple_ram_0/2
  simple_ram_0/1 -> rd_data/1
  rd_address/1 -> simple_ram_0/4
  wr_data/1 -> simple_ram_0/1
  wr_addr/1 -> wr_address/1
  wr_en/1 -> simple_ram_0/3
  rd_addr/1 -> rd_address/1

== system gm_hybrid_lht_vnl/Hybrid LHT/Hybrid LHT Accumulator/Accumulator with Switches/Accumulator_instance13/Block RAM/Simple Dual Port RAM Generator ==
  wr_data : Inport  OutDataTypeStr=fixdt(0, 36, 0)  PortDimensions=1  SampleTime=8.33333333333333e-09
  wr_addr : Inport  Port=2  OutDataTypeStr=fixdt(0, 9, 0)  PortDimensions=1  SampleTime=8.33333333333333e-09
  wr_en : Inport  Port=3  OutDataTypeStr=boolean  PortDimensions=1  SampleTime=8.33333333333333e-09
  rd_addr : Inport  Port=4  OutDataTypeStr=fixdt(0, 9, 0)  PortDimensions=1  SampleTime=8.33333333333333e-09
  rd_address : hdlsllib/Logic and Bit Operations/Bit Slice  lidx=8  ridx=0
      settings: SourceProductName=Simulink  SourceProductBaseCode=SL
  simple_ram_0 : hdlsllib/HDL RAMs/Simple Dual Port RAM  ram_size=9
      settings: SourceProductName=Simulink  SourceProductBaseCode=SL
  wr_address : hdlsllib/Logic and Bit Operations/Bit Slice  lidx=8  ridx=0
      settings: SourceProductName=Simulink  SourceProductBaseCode=SL
  rd_data : Outport
  wires:
  wr_address/1 -> simple_ram_0/2
  simple_ram_0/1 -> rd_data/1
  rd_address/1 -> simple_ram_0/4
  wr_data/1 -> simple_ram_0/1
  wr_addr/1 -> wr_address/1
  wr_en/1 -> simple_ram_0/3
  rd_addr/1 -> rd_address/1

== system gm_hybrid_lht_vnl/Hybrid LHT/Hybrid LHT Accumulator/Accumulator with Switches/Accumulator_instance14/Block RAM/Simple Dual Port RAM Generator ==
  wr_data : Inport  OutDataTypeStr=fixdt(0, 36, 0)  PortDimensions=1  SampleTime=8.33333333333333e-09
  wr_addr : Inport  Port=2  OutDataTypeStr=fixdt(0, 9, 0)  PortDimensions=1  SampleTime=8.33333333333333e-09
  wr_en : Inport  Port=3  OutDataTypeStr=boolean  PortDimensions=1  SampleTime=8.33333333333333e-09
  rd_addr : Inport  Port=4  OutDataTypeStr=fixdt(0, 9, 0)  PortDimensions=1  SampleTime=8.33333333333333e-09
  rd_address : hdlsllib/Logic and Bit Operations/Bit Slice  lidx=8  ridx=0
      settings: SourceProductName=Simulink  SourceProductBaseCode=SL
  simple_ram_0 : hdlsllib/HDL RAMs/Simple Dual Port RAM  ram_size=9
      settings: SourceProductName=Simulink  SourceProductBaseCode=SL
  wr_address : hdlsllib/Logic and Bit Operations/Bit Slice  lidx=8  ridx=0
      settings: SourceProductName=Simulink  SourceProductBaseCode=SL
  rd_data : Outport
  wires:
  wr_address/1 -> simple_ram_0/2
  simple_ram_0/1 -> rd_data/1
  rd_address/1 -> simple_ram_0/4
  wr_data/1 -> simple_ram_0/1
  wr_addr/1 -> wr_address/1
  wr_en/1 -> simple_ram_0/3
  rd_addr/1 -> rd_address/1

== system gm_hybrid_lht_vnl/Hybrid LHT/Hybrid LHT Accumulator/Accumulator with Switches/Accumulator_instance15/Block RAM/Simple Dual Port RAM Generator ==
  wr_data : Inport  OutDataTypeStr=fixdt(0, 36, 0)  PortDimensions=1  SampleTime=8.33333333333333e-09
  wr_addr : Inport  Port=2  OutDataTypeStr=fixdt(0, 9, 0)  PortDimensions=1  SampleTime=8.33333333333333e-09
  wr_en : Inport  Port=3  OutDataTypeStr=boolean  PortDimensions=1  SampleTime=8.33333333333333e-09
  rd_addr : Inport  Port=4  OutDataTypeStr=fixdt(0, 9, 0)  PortDimensions=1  SampleTime=8.33333333333333e-09
  rd_address : hdlsllib/Logic and Bit Operations/Bit Slice  lidx=8  ridx=0
      settings: SourceProductName=Simulink  SourceProductBaseCode=SL
  simple_ram_0 : hdlsllib/HDL RAMs/Simple Dual Port RAM  ram_size=9
      settings: SourceProductName=Simulink  SourceProductBaseCode=SL
  wr_address : hdlsllib/Logic and Bit Operations/Bit Slice  lidx=8  ridx=0
      settings: SourceProductName=Simulink  SourceProductBaseCode=SL
  rd_data : Outport
  wires:
  wr_address/1 -> simple_ram_0/2
  simple_ram_0/1 -> rd_data/1
  rd_address/1 -> simple_ram_0/4
  wr_data/1 -> simple_ram_0/1
  wr_addr/1 -> wr_address/1
  wr_en/1 -> simple_ram_0/3
  rd_addr/1 -> rd_address/1

== system gm_hybrid_lht_vnl/Hybrid LHT/Hybrid LHT Accumulator/Accumulator with Switches/Accumulator_instance16/Block RAM/Simple Dual Port RAM Generator ==
  wr_data : Inport  OutDataTypeStr=fixdt(0, 36, 0)  PortDimensions=1  SampleTime=8.33333333333333e-09
  wr_addr : Inport  Port=2  OutDataTypeStr=fixdt(0, 9, 0)  PortDimensions=1  SampleTime=8.33333333333333e-09
  wr_en : Inport  Port=3  OutDataTypeStr=boolean  PortDimensions=1  SampleTime=8.33333333333333e-09
  rd_addr : Inport  Port=4  OutDataTypeStr=fixdt(0, 9, 0)  PortDimensions=1  SampleTime=8.33333333333333e-09
  rd_address : hdlsllib/Logic and Bit Operations/Bit Slice  lidx=8  ridx=0
      settings: SourceProductName=Simulink  SourceProductBaseCode=SL
  simple_ram_0 : hdlsllib/HDL RAMs/Simple Dual Port RAM  ram_size=9
      settings: SourceProductName=Simulink  SourceProductBaseCode=SL
  wr_address : hdlsllib/Logic and Bit Operations/Bit Slice  lidx=8  ridx=0
      settings: SourceProductName=Simulink  SourceProductBaseCode=SL
  rd_data : Outport
  wires:
  wr_address/1 -> simple_ram_0/2
  simple_ram_0/1 -> rd_data/1
  rd_address/1 -> simple_ram_0/4
  wr_data/1 -> simple_ram_0/1
  wr_addr/1 -> wr_address/1
  wr_en/1 -> simple_ram_0/3
  rd_addr/1 -> rd_address/1

== system gm_hybrid_lht_vnl/Hybrid LHT/Hybrid LHT Accumulator/Accumulator with Switches/Accumulator_instance17/Block RAM/Simple Dual Port RAM Generator ==
  wr_data : Inport  OutDataTypeStr=fixdt(0, 36, 0)  PortDimensions=1  SampleTime=8.33333333333333e-09
  wr_addr : Inport  Port=2  OutDataTypeStr=fixdt(0, 9, 0)  PortDimensions=1  SampleTime=8.33333333333333e-09
  wr_en : Inport  Port=3  OutDataTypeStr=boolean  PortDimensions=1  SampleTime=8.33333333333333e-09
  rd_addr : Inport  Port=4  OutDataTypeStr=fixdt(0, 9, 0)  PortDimensions=1  SampleTime=8.33333333333333e-09
  rd_address : hdlsllib/Logic and Bit Operations/Bit Slice  lidx=8  ridx=0
      settings: SourceProductName=Simulink  SourceProductBaseCode=SL
  simple_ram_0 : hdlsllib/HDL RAMs/Simple Dual Port RAM  ram_size=9
      settings: SourceProductName=Simulink  SourceProductBaseCode=SL
  wr_address : hdlsllib/Logic and Bit Operations/Bit Slice  lidx=8  ridx=0
      settings: SourceProductName=Simulink  SourceProductBaseCode=SL
  rd_data : Outport
  wires:
  wr_address/1 -> simple_ram_0/2
  simple_ram_0/1 -> rd_data/1
  rd_address/1 -> simple_ram_0/4
  wr_data/1 -> simple_ram_0/1
  wr_addr/1 -> wr_address/1
  wr_en/1 -> simple_ram_0/3
  rd_addr/1 -> rd_address/1

== system gm_hybrid_lht_vnl/Hybrid LHT/Hybrid LHT Accumulator/Accumulator with Switches/Accumulator_instance18/Block RAM/Simple Dual Port RAM Generator ==
  wr_data : Inport  OutDataTypeStr=fixdt(0, 36, 0)  PortDimensions=1  SampleTime=8.33333333333333e-09
  wr_addr : Inport  Port=2  OutDataTypeStr=fixdt(0, 9, 0)  PortDimensions=1  SampleTime=8.33333333333333e-09
  wr_en : Inport  Port=3  OutDataTypeStr=boolean  PortDimensions=1  SampleTime=8.33333333333333e-09
  rd_addr : Inport  Port=4  OutDataTypeStr=fixdt(0, 9, 0)  PortDimensions=1  SampleTime=8.33333333333333e-09
  rd_address : hdlsllib/Logic and Bit Operations/Bit Slice  lidx=8  ridx=0
      settings: SourceProductName=Simulink  SourceProductBaseCode=SL
  simple_ram_0 : hdlsllib/HDL RAMs/Simple Dual Port RAM  ram_size=9
      settings: SourceProductName=Simulink  SourceProductBaseCode=SL
  wr_address : hdlsllib/Logic and Bit Operations/Bit Slice  lidx=8  ridx=0
      settings: SourceProductName=Simulink  SourceProductBaseCode=SL
  rd_data : Outport
  wires:
  wr_address/1 -> simple_ram_0/2
  simple_ram_0/1 -> rd_data/1
  rd_address/1 -> simple_ram_0/4
  wr_data/1 -> simple_ram_0/1
  wr_addr/1 -> wr_address/1
  wr_en/1 -> simple_ram_0/3
  rd_addr/1 -> rd_address/1

== system gm_hybrid_lht_vnl/Hybrid LHT/Hybrid LHT Accumulator/Accumulator with Switches/Accumulator_instance19/Block RAM/Simple Dual Port RAM Generator ==
  wr_data : Inport  OutDataTypeStr=fixdt(0, 36, 0)  PortDimensions=1  SampleTime=8.33333333333333e-09
  wr_addr : Inport  Port=2  OutDataTypeStr=fixdt(0, 9, 0)  PortDimensions=1  SampleTime=8.33333333333333e-09
  wr_en : Inport  Port=3  OutDataTypeStr=boolean  PortDimensions=1  SampleTime=8.33333333333333e-09
  rd_addr : Inport  Port=4  OutDataTypeStr=fixdt(0, 9, 0)  PortDimensions=1  SampleTime=8.33333333333333e-09
  rd_address : hdlsllib/Logic and Bit Operations/Bit Slice  lidx=8  ridx=0
      settings: SourceProductName=Simulink  SourceProductBaseCode=SL
  simple_ram_0 : hdlsllib/HDL RAMs/Simple Dual Port RAM  ram_size=9
      settings: SourceProductName=Simulink  SourceProductBaseCode=SL
  wr_address : hdlsllib/Logic and Bit Operations/Bit Slice  lidx=8  ridx=0
      settings: SourceProductName=Simulink  SourceProductBaseCode=SL
  rd_data : Outport
  wires:
  wr_address/1 -> simple_ram_0/2
  simple_ram_0/1 -> rd_data/1
  rd_address/1 -> simple_ram_0/4
  wr_data/1 -> simple_ram_0/1
  wr_addr/1 -> wr_address/1
  wr_en/1 -> simple_ram_0/3
  rd_addr/1 -> rd_address/1

== system gm_hybrid_lht_vnl/Hybrid LHT/Hybrid LHT Accumulator/Accumulator with Switches/Accumulator_instance2/Block RAM/Simple Dual Port RAM Generator ==
  wr_data : Inport  OutDataTypeStr=fixdt(0, 36, 0)  PortDimensions=1  SampleTime=8.33333333333333e-09
  wr_addr : Inport  Port=2  OutDataTypeStr=fixdt(0, 9, 0)  PortDimensions=1  SampleTime=8.33333333333333e-09
  wr_en : Inport  Port=3  OutDataTypeStr=boolean  PortDimensions=1  SampleTime=8.33333333333333e-09
  rd_addr : Inport  Port=4  OutDataTypeStr=fixdt(0, 9, 0)  PortDimensions=1  SampleTime=8.33333333333333e-09
  rd_address : hdlsllib/Logic and Bit Operations/Bit Slice  lidx=8  ridx=0
      settings: SourceProductName=Simulink  SourceProductBaseCode=SL
  simple_ram_0 : hdlsllib/HDL RAMs/Simple Dual Port RAM  ram_size=9
      settings: SourceProductName=Simulink  SourceProductBaseCode=SL
  wr_address : hdlsllib/Logic and Bit Operations/Bit Slice  lidx=8  ridx=0
      settings: SourceProductName=Simulink  SourceProductBaseCode=SL
  rd_data : Outport
  wires:
  wr_address/1 -> simple_ram_0/2
  simple_ram_0/1 -> rd_data/1
  rd_address/1 -> simple_ram_0/4
  wr_data/1 -> simple_ram_0/1
  wr_addr/1 -> wr_address/1
  wr_en/1 -> simple_ram_0/3
  rd_addr/1 -> rd_address/1

== system gm_hybrid_lht_vnl/Hybrid LHT/Hybrid LHT Accumulator/Accumulator with Switches/Accumulator_instance20/Block RAM/Simple Dual Port RAM Generator ==
  wr_data : Inport  OutDataTypeStr=fixdt(0, 36, 0)  PortDimensions=1  SampleTime=8.33333333333333e-09
  wr_addr : Inport  Port=2  OutDataTypeStr=fixdt(0, 9, 0)  PortDimensions=1  SampleTime=8.33333333333333e-09
  wr_en : Inport  Port=3  OutDataTypeStr=boolean  PortDimensions=1  SampleTime=8.33333333333333e-09
  rd_addr : Inport  Port=4  OutDataTypeStr=fixdt(0, 9, 0)  PortDimensions=1  SampleTime=8.33333333333333e-09
  rd_address : hdlsllib/Logic and Bit Operations/Bit Slice  lidx=8  ridx=0
      settings: SourceProductName=Simulink  SourceProductBaseCode=SL
  simple_ram_0 : hdlsllib/HDL RAMs/Simple Dual Port RAM  ram_size=9
      settings: SourceProductName=Simulink  SourceProductBaseCode=SL
  wr_address : hdlsllib/Logic and Bit Operations/Bit Slice  lidx=8  ridx=0
      settings: SourceProductName=Simulink  SourceProductBaseCode=SL
  rd_data : Outport
  wires:
  wr_address/1 -> simple_ram_0/2
  simple_ram_0/1 -> rd_data/1
  rd_address/1 -> simple_ram_0/4
  wr_data/1 -> simple_ram_0/1
  wr_addr/1 -> wr_address/1
  wr_en/1 -> simple_ram_0/3
  rd_addr/1 -> rd_address/1

== system gm_hybrid_lht_vnl/Hybrid LHT/Hybrid LHT Accumulator/Accumulator with Switches/Accumulator_instance21/Block RAM/Simple Dual Port RAM Generator ==
  wr_data : Inport  OutDataTypeStr=fixdt(0, 36, 0)  PortDimensions=1  SampleTime=8.33333333333333e-09
  wr_addr : Inport  Port=2  OutDataTypeStr=fixdt(0, 9, 0)  PortDimensions=1  SampleTime=8.33333333333333e-09
  wr_en : Inport  Port=3  OutDataTypeStr=boolean  PortDimensions=1  SampleTime=8.33333333333333e-09
  rd_addr : Inport  Port=4  OutDataTypeStr=fixdt(0, 9, 0)  PortDimensions=1  SampleTime=8.33333333333333e-09
  rd_address : hdlsllib/Logic and Bit Operations/Bit Slice  lidx=8  ridx=0
      settings: SourceProductName=Simulink  SourceProductBaseCode=SL
  simple_ram_0 : hdlsllib/HDL RAMs/Simple Dual Port RAM  ram_size=9
      settings: SourceProductName=Simulink  SourceProductBaseCode=SL
  wr_address : hdlsllib/Logic and Bit Operations/Bit Slice  lidx=8  ridx=0
      settings: SourceProductName=Simulink  SourceProductBaseCode=SL
  rd_data : Outport
  wires:
  wr_address/1 -> simple_ram_0/2
  simple_ram_0/1 -> rd_data/1
  rd_address/1 -> simple_ram_0/4
  wr_data/1 -> simple_ram_0/1
  wr_addr/1 -> wr_address/1
  wr_en/1 -> simple_ram_0/3
  rd_addr/1 -> rd_address/1

== system gm_hybrid_lht_vnl/Hybrid LHT/Hybrid LHT Accumulator/Accumulator with Switches/Accumulator_instance22/Block RAM/Simple Dual Port RAM Generator ==
  wr_data : Inport  OutDataTypeStr=fixdt(0, 36, 0)  PortDimensions=1  SampleTime=8.33333333333333e-09
  wr_addr : Inport  Port=2  OutDataTypeStr=fixdt(0, 9, 0)  PortDimensions=1  SampleTime=8.33333333333333e-09
  wr_en : Inport  Port=3  OutDataTypeStr=boolean  PortDimensions=1  SampleTime=8.33333333333333e-09
  rd_addr : Inport  Port=4  OutDataTypeStr=fixdt(0, 9, 0)  PortDimensions=1  SampleTime=8.33333333333333e-09
  rd_address : hdlsllib/Logic and Bit Operations/Bit Slice  lidx=8  ridx=0
      settings: SourceProductName=Simulink  SourceProductBaseCode=SL
  simple_ram_0 : hdlsllib/HDL RAMs/Simple Dual Port RAM  ram_size=9
      settings: SourceProductName=Simulink  SourceProductBaseCode=SL
  wr_address : hdlsllib/Logic and Bit Operations/Bit Slice  lidx=8  ridx=0
      settings: SourceProductName=Simulink  SourceProductBaseCode=SL
  rd_data : Outport
  wires:
  wr_address/1 -> simple_ram_0/2
  simple_ram_0/1 -> rd_data/1
  rd_address/1 -> simple_ram_0/4
  wr_data/1 -> simple_ram_0/1
  wr_addr/1 -> wr_address/1
  wr_en/1 -> simple_ram_0/3
  rd_addr/1 -> rd_address/1

== system gm_hybrid_lht_vnl/Hybrid LHT/Hybrid LHT Accumulator/Accumulator with Switches/Accumulator_instance23/Block RAM/Simple Dual Port RAM Generator ==
  wr_data : Inport  OutDataTypeStr=fixdt(0, 36, 0)  PortDimensions=1  SampleTime=8.33333333333333e-09
  wr_addr : Inport  Port=2  OutDataTypeStr=fixdt(0, 9, 0)  PortDimensions=1  SampleTime=8.33333333333333e-09
  wr_en : Inport  Port=3  OutDataTypeStr=boolean  PortDimensions=1  SampleTime=8.33333333333333e-09
  rd_addr : Inport  Port=4  OutDataTypeStr=fixdt(0, 9, 0)  PortDimensions=1  SampleTime=8.33333333333333e-09
  rd_address : hdlsllib/Logic and Bit Operations/Bit Slice  lidx=8  ridx=0
      settings: SourceProductName=Simulink  SourceProductBaseCode=SL
  simple_ram_0 : hdlsllib/HDL RAMs/Simple Dual Port RAM  ram_size=9
      settings: SourceProductName=Simulink  SourceProductBaseCode=SL
  wr_address : hdlsllib/Logic and Bit Operations/Bit Slice  lidx=8  ridx=0
      settings: SourceProductName=Simulink  SourceProductBaseCode=SL
  rd_data : Outport
  wires:
  wr_address/1 -> simple_ram_0/2
  simple_ram_0/1 -> rd_data/1
  rd_address/1 -> simple_ram_0/4
  wr_data/1 -> simple_ram_0/1
  wr_addr/1 -> wr_address/1
  wr_en/1 -> simple_ram_0/3
  rd_addr/1 -> rd_address/1
